simulink model "Model_vmaRHTS_R2019b_statespace"  (R2023a)
settings: Solver=ode4  StartTime=0.0  StopTime=100  FixedStep=dt  RelTol=1e-3
undefined symbols (not defined in the file): a0, a1, a2, a3, a4, a5, a6, a7, A_cplant, A_G1, A_Gpd, AgN, alpha1, alpha2, B_cplant, B_G1, B_Gpd, C_cplant, C_G1, C_Gpd, C_phys_5dof, CNrt, Cren, D_cplant, D_G1, D_Gpd, Ds, dt, dv1, dv2, EQ_intensity, EQ_sw, FN, G1, Gcld, Gd1, Gnd_ss, Hs1, Hs2, j1, j2, k3, k4, k6, K_phys_5dof, KNbar_inv, Koo, Kot, Kren, lN, M_phys_5dof, MNrt, Mren, RNbar
libraries: slpidlib x4, sldrtlib x1, dspsrcs4 x1
settings Model: Creator=icu327  LastModifiedBy=liangyu
settings SolverCC: AlgebraicLoopSolver=TrustRegion
settings DataIOCC: SaveFormat=Array  ReturnWorkspaceOutputs=off
settings DebuggingCC: UnconnectedInputMsg=warning  UnconnectedOutputMsg=warning  UnconnectedLineMsg=warning  ArithmeticOperatorsInVariantConditions=warning
settings HardwareCC: ProdBitPerLong=64  ProdHWDeviceType=Intel->x86-64 (Linux 64)
settings ModelReferenceCC: EnableRefExpFcnMdlSchedulingChecks=on
settings SFSimCC: CustomCodeUndefinedFunction=UseInterfaceOnly
settings RTWCC: Description=Simulink Desktop Real-Time  SystemTargetFile=sldrt.tlc  TemplateMakefile=sldrt.tmf  RTWCompilerOptimization=on
settings CodeAppCC: MaxIdLength=95  StateflowObjectComments=on
settings SimulinkDesktopRealTimeCC: TargetLibSuffix=_sldrt.a  TargetPreCompLibLocation=C:\Program Files\MATLAB\R2023a\toolbox\sldrt\lib\win64

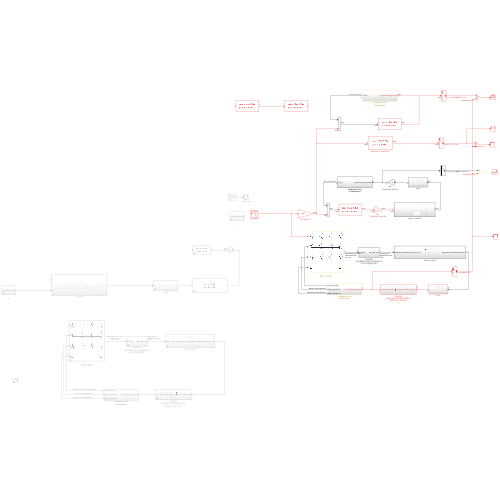
[thumbnail: Simulink's stored preview of the top-level diagram]
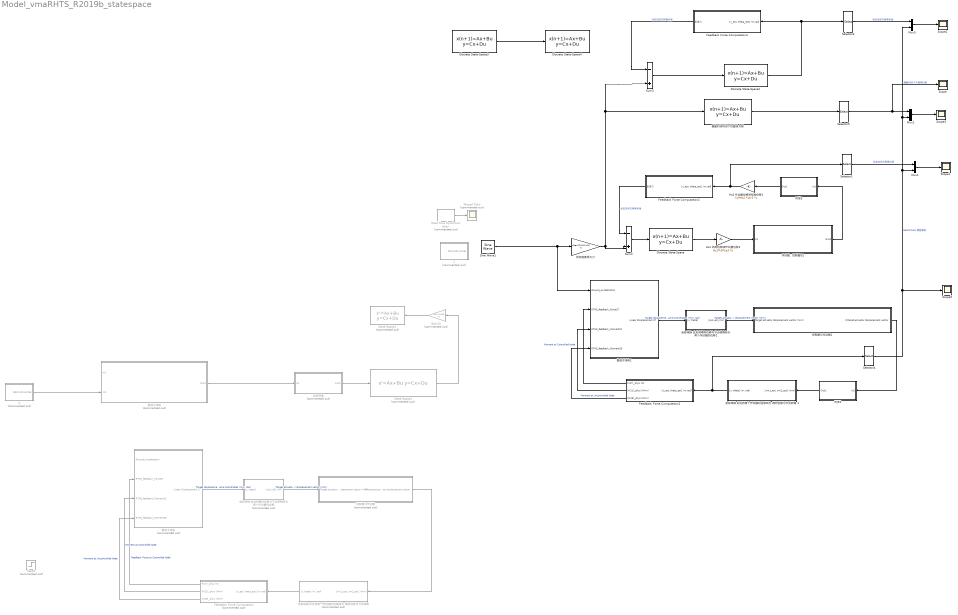
== system Model_vmaRHTS_R2019b_statespace ==
  " 2" : Subsystem  Commented=on
  " 4" : Subsystem  Commented=on
  " 数值子结构" : Subsystem  Commented=on
      mask Display: image('$imagefile'); % Use "Edit Image" on toolstrip to change.
  " 数值子结构1" : Subsystem
      mask Display: image('$imagefile'); % Use "Edit Image" on toolstrip to change.
  Discrete State-Space : DiscreteStateSpace  A=Gnd_ss.A  B=Gnd_ss.B  C=Gnd_ss.C  D=Gnd_ss.D  SampleTime=-1
  Discrete State-Space2 : DiscreteStateSpace  A=Gd1.A  B=Gd1.B  C=Gd1.C  D=Gd1.D  SampleTime=-1
  Discrete State-Space3 : DiscreteStateSpace  A=Gnd_ss.A  B=Gnd_ss.B  C=Gnd_ss.C  D=Gnd_ss.D  SampleTime=-1
  Discrete State-Space4 : DiscreteStateSpace  A=Ds.A  B=Ds.B  C=Ds.C  D=Ds.D  SampleTime=-1
  Feedback Force Computation : Subsystem  Commented=on
  Feedback Force Computation1 : Subsystem
  Feedback Force Computation2 : Subsystem
  Feedback Force Computation4 : Subsystem
  Gain10 : Gain  Commented=on  Gain=Hs2./1000  Multiplication=Matrix(K*u)
  Hs1 结构位移转作动器位移2 : Gain  Gain=Hs1*k6*1e3  Multiplication=Matrix(K*u)
  Hs2 作动器位移转结构位移1 : Gain  Gain=k4*Hs2.*1e-3  Multiplication=Matrix(K*u)
  Missed Ticks : Scope  Commented=on
  Mux1 : Mux  Inputs=2
  Mux2 : Mux  Inputs=2
  Mux3 : Mux  Inputs=2
  Real-Time Synchronization : sldrtlib/Real-Time Synchronization  Commented=on  SampleTime=dt  MaxMissedTicks=10000  ShowMissedTicks=on  YieldWhenWaiting=off
  Scope{,1..3,5} (5 alike) : Scope
  Selector1 : Selector  InputPortWidth=5  IndexOptions=Index vector (dialog)  Indices=[1]  OutputSizes=1
  Selector3 : Selector  InputPortWidth=5  IndexOptions=Index vector (dialog)  Indices=[1]  OutputSizes=1
  Selector4 : Selector  InputPortWidth=2  IndexOptions=Index vector (dialog)  Indices=[1]  OutputSizes=1
  Selector5 : Selector  InputPortWidth=5  IndexOptions=Index vector (dialog)  Indices=[1]  OutputSizes=1
  Sine Wave1 : dspsrcs4/Sine Wave  Amplitude=1  Frequency=1  Phase=0  SampleMode=Discrete  OutComplex=Real  CompMethod=Trigonometric fcn  TableSize=Speed  SampleTime=dt  SamplesPerFrame=1  ResetState=Restart at time zero  OutputFrames=off  dataType=double  wordLen=16  udDataType=sfix(16)  fracBitsMode=Best precision  numFracBits=15  OutDataTypeStr=double  LastOutDataTypeStr=double
  State-Space2 : StateSpace  Commented=on  A=A_G1  B=B_G1  C=C_G1  D=D_G1  InitialCondition=0
  State-Space3 : StateSpace  Commented=on  A=A_Gpd  B=B_Gpd  C=C_Gpd  D=D_Gpd  InitialCondition=0
  Step5 : Step  Commented=on  SampleTime=0
  Sum2 : Sum  Inputs=-|+
  Sum3 : Sum  Inputs=-|+
  作动器、控制器G1 : Subsystem
  坐标转换 : Subsystem  Commented=on
  "坐标转换 此处将两个作动器的位移转为 横向位移与节点转角 " : Subsystem  Commented=on
  坐标转换 此处将两个作动器的位移转为 横向位移与节点转角 1 : Subsystem
  坐标转换 此处将横向位移与节点转角转为 两个作动器的位移 : Subsystem  Commented=on
  坐标转换 此处将横向位移与节点转角转为 两个作动器的位移1 : Subsystem
  将加速度转为力 : Gain  Gain=-Mren*[1;0;1;1;0]  Multiplication=Matrix(K*u)
  控制器与作动器 : Subsystem  Commented=on
  控制器与作动器1 : Subsystem
  数值子结构 : Subsystem  Commented=on
  时滞2 : Subsystem
  时滞3 : Subsystem
  离散时间时间下的整体方程 : DiscreteStateSpace  A=Gcld.A  B=Gcld.B  C=Gcld.C  D=Gcld.D  SampleTime=-1
  wires:
  Feedback Force Computation/1(F(27)_phys (N)) -> " 数值子结构"/2(RTHS_feedback_Force27)  "Feedback Force at Controlled Node"
  Feedback Force Computation/3(M(29)_phys (N*m)) -> " 数值子结构"/4(RTHS_feedback_Moment29)  "Moment at Uncontrolled Node"
  "坐标转换 此处将两个作动器的位移转为 横向位移与节点转角 "/1("[x, theta] (m, rad)") -> Feedback Force Computation/1("[x_est, theta_est] (m,rad)")
  " 数值子结构"/1(Linear Displacement 27) -> 坐标转换 此处将横向位移与节点转角转为 两个作动器的位移/1("[x, theta]")  "Target displacement vector Frame coordinates (mm, rad)"
  Feedback Force Computation/2(M(21)_phys (N*m)) -> " 数值子结构"/3(RTHS_feedback_Moment21)  "Moment at Controlled Node"
  坐标转换 此处将横向位移与节点转角转为 两个作动器的位移/1("[xa1,xa2] mm") -> 控制器与作动器/1(Target actuator displacement vector (mm))  "Target actuator displacement vector (mm)"
  控制器与作动器/1(Filtered actuator displacement vector) -> "坐标转换 此处将两个作动器的位移转为 横向位移与节点转角 "/1("[xm1_est, xm2_est] (mm)")
  " 数值子结构1"/1(Linear Displacement 27) -> 坐标转换 此处将横向位移与节点转角转为 两个作动器的位移1/1("[x, theta]")  "Target displacement vector Frame coordinates (mm, rad)"
  坐标转换 此处将横向位移与节点转角转为 两个作动器的位移1/1("[xa1,xa2] mm") -> 控制器与作动器1/1(Target actuator displacement vector (mm))  "Target actuator displacement vector (mm)"
  Gain10/1 -> State-Space3/1
  State-Space2/1 -> Gain10/1
  " 4"/1(GROUND ACCEL) -> 数值子结构/2(In2)
  数值子结构/1(Out1) -> 坐标转换/1(In1)
  坐标转换/1(Out1) -> State-Space2/1
  Real-Time Synchronization/1 -> Missed Ticks/1
  Sine Wave1/1 -> " 数值子结构1"/1(Ground_Acceleration), 将加速度转为力/1
  Feedback Force Computation1/1(F(27)_phys (N)) -> " 数值子结构1"/2(RTHS_feedback_Force27)
  Feedback Force Computation1/2(M(21)_phys (N*m)) -> " 数值子结构1"/3(RTHS_feedback_Moment21)  "Moment at Controlled Node"
  Feedback Force Computation1/3(M(29)_phys (N*m)) -> " 数值子结构1"/4(RTHS_feedback_Moment29)  "Moment at Uncontrolled Node"
  Mux2/1 -> Scope3/1
  离散时间时间下的整体方程/1 -> Selector5/1
  Selector5/1 -> Scope/1, Mux2/1  "离散时间下方程等价版"
  控制器与作动器1/1(Filtered actuator displacement vector) -> 时滞2/1(In1)
  坐标转换 此处将两个作动器的位移转为 横向位移与节点转角 1/1("[x, theta] (m, rad)") -> Feedback Force Computation1/1("[x_est, theta_est] (m,rad)"), Selector4/1
  时滞2/1(Out1) -> 坐标转换 此处将两个作动器的位移转为 横向位移与节点转角 1/1("[xm1_est, xm2_est] (mm)")
  将加速度转为力/1 -> Sum3/2, 离散时间时间下的整体方程/1, Sum2/2
  作动器、控制器G1/1(Out1) -> 时滞3/1(In1)
  Feedback Force Computation2/1(反馈力) -> Sum2/1  "状态空间方程等价版"
  Hs2 作动器位移转结构位移1/1 -> Selector1/1, Feedback Force Computation2/1("[x_est, theta_est] (m,rad)")
  Discrete State-Space/1 -> Hs1 结构位移转作动器位移2/1
  时滞3/1(Out1) -> Hs2 作动器位移转结构位移1/1
  Sum2/1 -> Discrete State-Space/1
  Hs1 结构位移转作动器位移2/1 -> 作动器、控制器G1/1(In1)
  Selector1/1 -> Mux1/1  "状态空间方程等价版"
  Mux1/1 -> Scope1/1
  Mux3/1 -> Scope2/1
  Sum3/1 -> Discrete State-Space2/1
  Selector4/1 -> Mux3/2, Mux2/2, Mux1/2, Scope5/1  "benchmark模型原版"
  Selector3/1 -> Mux3/1  "状态空间方程等价版"
  Feedback Force Computation4/1(反馈力) -> Sum3/1  "状态空间方程等价版"
  Discrete State-Space2/1 -> Feedback Force Computation4/1("[x_est, theta_est] (m,rad)"), Selector3/1
  Discrete State-Space3/1 -> Discrete State-Space4/1

== system Model_vmaRHTS_R2019b_statespace/ 2 ==
  note: Benchmark Control Problem for
      | Multi-axial Real-time Hybrid Simulation
      | Ground Acceleration
  Clock : Clock
  EQ scaling factor : Gain  Gain=EQ_intensity  Multiplication=Matrix(K*u)
  GROUND ACCELERATION : ToWorkspace  VariableName=EQ_input  SampleTime=-1
      settings: Save2DSignal=2-D array (concatenate along first dimension)
  Ground motion record : Subsystem
  Multiport Switch : MultiPortSwitch  SaturateOnIntegerOverflow=off  InputSameDT=off
  SWITCH CONSTANT : Constant  Value=EQ_sw
  To Workspace : ToWorkspace  VariableName=t  SampleTime=dt
  GROUND ACCEL : Outport  VectorParamsAs1DForOutWhenUnconnected=off
  wires:
  Multiport Switch/1 -> EQ scaling factor/1
  EQ scaling factor/1 -> GROUND ACCELERATION/1, GROUND ACCEL/1
  Ground motion record/1(El Centro) -> Multiport Switch/2
  Ground motion record/2(Kobe) -> Multiport Switch/3
  Ground motion record/3(Morgan) -> Multiport Switch/4
  SWITCH CONSTANT/1 -> Multiport Switch/1
  Clock/1 -> To Workspace/1

== system Model_vmaRHTS_R2019b_statespace/ 4 ==
  note: Benchmark Control Problem for
      | Multi-axial Real-time Hybrid Simulation
      | Ground Acceleration
  Clock : Clock
  EQ scaling factor : Gain  Gain=EQ_intensity  Multiplication=Matrix(K*u)
  GROUND ACCELERATION : ToWorkspace  VariableName=EQ_input  SampleTime=-1
      settings: Save2DSignal=2-D array (concatenate along first dimension)
  Ground motion record : Subsystem
  Multiport Switch : MultiPortSwitch  SaturateOnIntegerOverflow=off  InputSameDT=off
  SWITCH CONSTANT : Constant  Value=EQ_sw
  To Workspace : ToWorkspace  VariableName=t  SampleTime=dt
  GROUND ACCEL : Outport  VectorParamsAs1DForOutWhenUnconnected=off
  wires:
  Multiport Switch/1 -> EQ scaling factor/1
  EQ scaling factor/1 -> GROUND ACCELERATION/1, GROUND ACCEL/1
  Ground motion record/1(El Centro) -> Multiport Switch/2
  Ground motion record/2(Kobe) -> Multiport Switch/3
  Ground motion record/3(Morgan) -> Multiport Switch/4
  SWITCH CONSTANT/1 -> Multiport Switch/1
  Clock/1 -> To Workspace/1

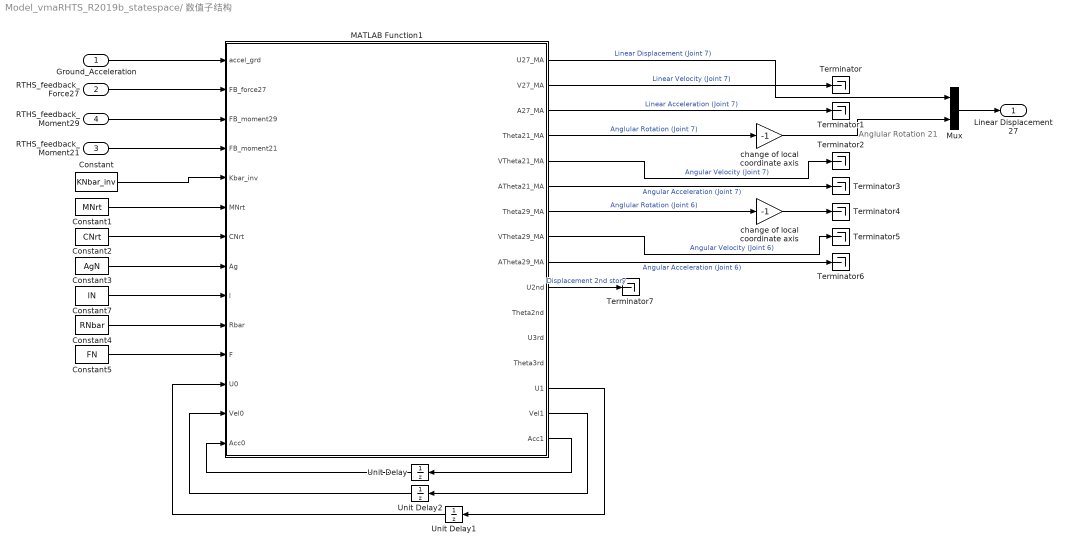
== system Model_vmaRHTS_R2019b_statespace/ 数值子结构 ==
  note: Anglular Rotation 21
  Ground_Acceleration : Inport
  RTHS_feedback_Force27 : Inport  Port=2
  RTHS_feedback_Moment21 : Inport  Port=3
  RTHS_feedback_Moment29 : Inport  Port=4
  Constant : Constant  Value=KNbar_inv  VectorParams1D=off
  Constant1 : Constant  Value=MNrt  VectorParams1D=off
  Constant2 : Constant  Value=CNrt  VectorParams1D=off
  Constant3 : Constant  Value=AgN  VectorParams1D=off
  Constant4 : Constant  Value=RNbar  VectorParams1D=off
  Constant5 : Constant  Value=FN  VectorParams1D=off
  Constant7 : Constant  Value=lN  VectorParams1D=off
  MATLAB Function1 : MATLAB Function  TreatAsAtomicUnit=on
  Mux : Mux  Inputs=2
  Terminator{,1..7} (8 alike) : Terminator
  Unit Delay : UnitDelay  SampleTime=-1  HasFrameUpgradeWarning=on
  Unit Delay1 : UnitDelay  SampleTime=-1  HasFrameUpgradeWarning=on
  Unit Delay2 : UnitDelay  SampleTime=-1  HasFrameUpgradeWarning=on
  change of local coordinate axis : Gain  Gain=-1
  "change of local coordinate axis  " : Gain  Gain=-1
  Linear Displacement 27 : Outport  VectorParamsAs1DForOutWhenUnconnected=off
  wires:
  Ground_Acceleration/1 -> MATLAB Function1/1(accel_grd)
  RTHS_feedback_Force27/1 -> MATLAB Function1/2(FB_force27)
  RTHS_feedback_Moment29/1 -> MATLAB Function1/3(FB_moment29)
  MATLAB Function1/1(U27_MA) -> Mux/1  "Linear Displacement (Joint 7)"
  MATLAB Function1/4(Theta21_MA) -> change of local coordinate axis/1  "Anglular Rotation (Joint 7)"
  Constant/1 -> MATLAB Function1/5(Kbar_inv)
  Constant1/1 -> MATLAB Function1/6(MNrt)
  Constant2/1 -> MATLAB Function1/7(CNrt)
  Constant3/1 -> MATLAB Function1/8(Ag)
  Constant7/1 -> MATLAB Function1/9(l)
  Constant4/1 -> MATLAB Function1/10(Rbar)
  Unit Delay1/1 -> MATLAB Function1/12(U0)
  Unit Delay2/1 -> MATLAB Function1/13(Vel0)
  Unit Delay/1 -> MATLAB Function1/14(Acc0)
  MATLAB Function1/15(Vel1) -> Unit Delay2/1
  MATLAB Function1/16(Acc1) -> Unit Delay/1
  MATLAB Function1/14(U1) -> Unit Delay1/1
  Constant5/1 -> MATLAB Function1/11(F)
  MATLAB Function1/2(V27_MA) -> Terminator/1  "Linear Velocity (Joint 7)"
  MATLAB Function1/3(A27_MA) -> Terminator1/1  "Linear Acceleration (Joint 7)"
  MATLAB Function1/5(VTheta21_MA) -> Terminator2/1  "Angular Velocity (Joint 7)"
  MATLAB Function1/6(ATheta21_MA) -> Terminator3/1  "Angular Acceleration (Joint 7)"
  MATLAB Function1/9(ATheta29_MA) -> Terminator6/1  "Angular Acceleration (Joint 6)"
  MATLAB Function1/8(VTheta29_MA) -> Terminator5/1  "Angular Velocity (Joint 6)"
  MATLAB Function1/7(Theta29_MA) -> "change of local coordinate axis  "/1  "Anglular Rotation (Joint 6)"
  RTHS_feedback_Moment21/1 -> MATLAB Function1/4(FB_moment21)
  change of local coordinate axis/1 -> Mux/2
  "change of local coordinate axis  "/1 -> Terminator4/1
  Mux/1 -> Linear Displacement 27/1
  MATLAB Function1/10(U2nd) -> Terminator7/1  "Displacement 2nd story"

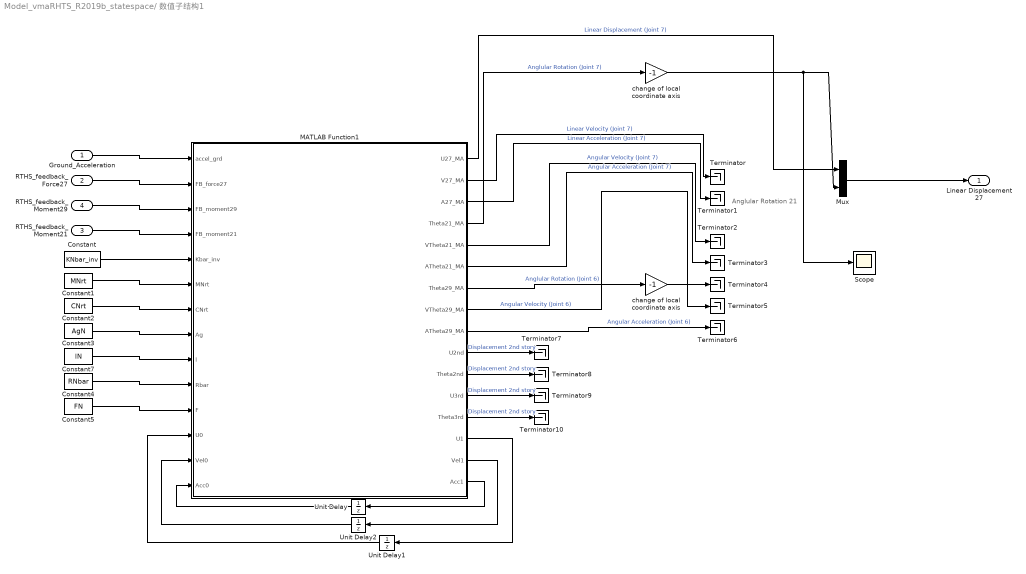
== system Model_vmaRHTS_R2019b_statespace/ 数值子结构1 ==
  note: Anglular Rotation 21
  Ground_Acceleration : Inport
  RTHS_feedback_Force27 : Inport  Port=2
  RTHS_feedback_Moment21 : Inport  Port=3
  RTHS_feedback_Moment29 : Inport  Port=4
  Constant : Constant  Value=KNbar_inv  VectorParams1D=off
  Constant1 : Constant  Value=MNrt  VectorParams1D=off
  Constant2 : Constant  Value=CNrt  VectorParams1D=off
  Constant3 : Constant  Value=AgN  VectorParams1D=off
  Constant4 : Constant  Value=RNbar  VectorParams1D=off
  Constant5 : Constant  Value=FN  VectorParams1D=off
  Constant7 : Constant  Value=lN  VectorParams1D=off
  MATLAB Function1 : MATLAB Function  TreatAsAtomicUnit=on
  Mux : Mux  Inputs=2
  Scope : Scope
  Terminator{,1..10} (11 alike) : Terminator
  Unit Delay : UnitDelay  SampleTime=-1  HasFrameUpgradeWarning=on
  Unit Delay1 : UnitDelay  SampleTime=-1  HasFrameUpgradeWarning=on
  Unit Delay2 : UnitDelay  SampleTime=-1  HasFrameUpgradeWarning=on
  change of local coordinate axis : Gain  Gain=-1
  "change of local coordinate axis  " : Gain  Gain=-1
  Linear Displacement 27 : Outport  VectorParamsAs1DForOutWhenUnconnected=off
  wires:
  Ground_Acceleration/1 -> MATLAB Function1/1(accel_grd)
  RTHS_feedback_Force27/1 -> MATLAB Function1/2(FB_force27)
  RTHS_feedback_Moment29/1 -> MATLAB Function1/3(FB_moment29)
  MATLAB Function1/1(U27_MA) -> Mux/1  "Linear Displacement (Joint 7)"
  MATLAB Function1/4(Theta21_MA) -> change of local coordinate axis/1  "Anglular Rotation (Joint 7)"
  Constant/1 -> MATLAB Function1/5(Kbar_inv)
  Constant1/1 -> MATLAB Function1/6(MNrt)
  Constant2/1 -> MATLAB Function1/7(CNrt)
  Constant3/1 -> MATLAB Function1/8(Ag)
  Constant7/1 -> MATLAB Function1/9(l)
  Constant4/1 -> MATLAB Function1/10(Rbar)
  Unit Delay1/1 -> MATLAB Function1/12(U0)
  Unit Delay2/1 -> MATLAB Function1/13(Vel0)
  Unit Delay/1 -> MATLAB Function1/14(Acc0)
  MATLAB Function1/15(Vel1) -> Unit Delay2/1
  MATLAB Function1/16(Acc1) -> Unit Delay/1
  MATLAB Function1/14(U1) -> Unit Delay1/1
  Constant5/1 -> MATLAB Function1/11(F)
  MATLAB Function1/2(V27_MA) -> Terminator/1  "Linear Velocity (Joint 7)"
  MATLAB Function1/3(A27_MA) -> Terminator1/1  "Linear Acceleration (Joint 7)"
  MATLAB Function1/5(VTheta21_MA) -> Terminator2/1  "Angular Velocity (Joint 7)"
  MATLAB Function1/6(ATheta21_MA) -> Terminator3/1  "Angular Acceleration (Joint 7)"
  MATLAB Function1/9(ATheta29_MA) -> Terminator6/1  "Angular Acceleration (Joint 6)"
  MATLAB Function1/8(VTheta29_MA) -> Terminator5/1  "Angular Velocity (Joint 6)"
  MATLAB Function1/7(Theta29_MA) -> "change of local coordinate axis  "/1  "Anglular Rotation (Joint 6)"
  RTHS_feedback_Moment21/1 -> MATLAB Function1/4(FB_moment21)
  change of local coordinate axis/1 -> Scope/1, Mux/2
  "change of local coordinate axis  "/1 -> Terminator4/1
  Mux/1 -> Linear Displacement 27/1
  MATLAB Function1/10(U2nd) -> Terminator7/1  "Displacement 2nd story"
  MATLAB Function1/11(Theta2nd) -> Terminator8/1  "Displacement 2nd story"
  MATLAB Function1/12(U3rd) -> Terminator9/1  "Displacement 2nd story"
  MATLAB Function1/13(Theta3rd) -> Terminator10/1  "Displacement 2nd story"

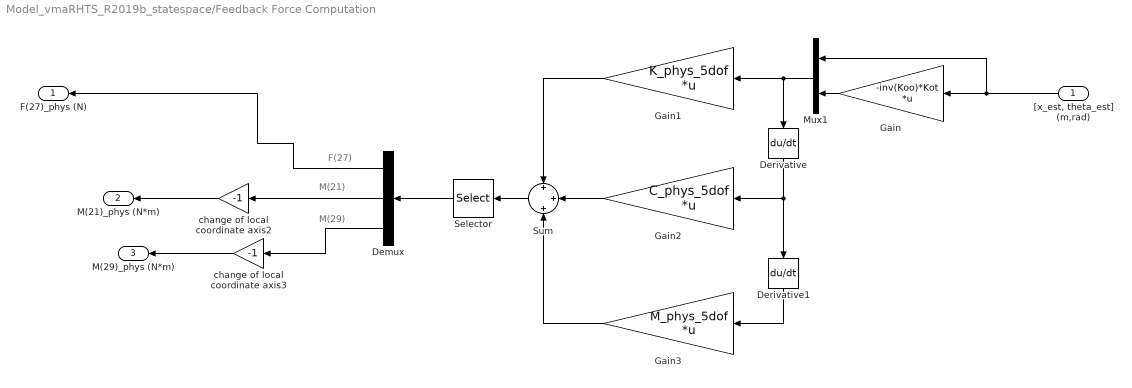
== system Model_vmaRHTS_R2019b_statespace/Feedback Force Computation ==
  note: F(27)
  note: M(21)
  note: M(29)
  "[x_est, theta_est] (m,rad)" : Inport
  Demux : Demux  Outputs=3
  Derivative : Derivative
  Derivative1 : Derivative
  Gain : Gain  Gain=-inv(Koo)*Kot  Multiplication=Matrix(K*u) (u vector)
  Gain1 : Gain  Gain=K_phys_5dof  Multiplication=Matrix(K*u) (u vector)
  Gain2 : Gain  Gain=C_phys_5dof  Multiplication=Matrix(K*u) (u vector)
  Gain3 : Gain  Gain=M_phys_5dof  Multiplication=Matrix(K*u) (u vector)
  Mux1 : Mux  Inputs=2
  Selector : Selector  InputPortWidth=5  IndexOptions=Index vector (dialog)  Indices=[1 2 3]  OutputSizes=1
  Sum : Sum  Inputs=+|+|+
  change of local coordinate axis2 : Gain  Gain=-1
  change of local coordinate axis3 : Gain  Gain=-1
  F(27)_phys (N) : Outport  VectorParamsAs1DForOutWhenUnconnected=off
  M(21)_phys (N*m) : Outport  Port=2  VectorParamsAs1DForOutWhenUnconnected=off
  M(29)_phys (N*m) : Outport  Port=3  VectorParamsAs1DForOutWhenUnconnected=off
  wires:
  Gain/1 -> Mux1/2
  Derivative1/1 -> Gain3/1
  Gain2/1 -> Sum/2
  Derivative/1 -> Gain2/1, Derivative1/1
  Gain1/1 -> Sum/1
  "[x_est, theta_est] (m,rad)"/1 -> Gain/1, Mux1/1
  Demux/1 -> F(27)_phys (N)/1
  Sum/1 -> Selector/1
  Selector/1 -> Demux/1
  Gain3/1 -> Sum/3
  Demux/2 -> change of local coordinate axis2/1
  Demux/3 -> change of local coordinate axis3/1
  Mux1/1 -> Derivative/1, Gain1/1
  change of local coordinate axis2/1 -> M(21)_phys (N*m)/1
  change of local coordinate axis3/1 -> M(29)_phys (N*m)/1

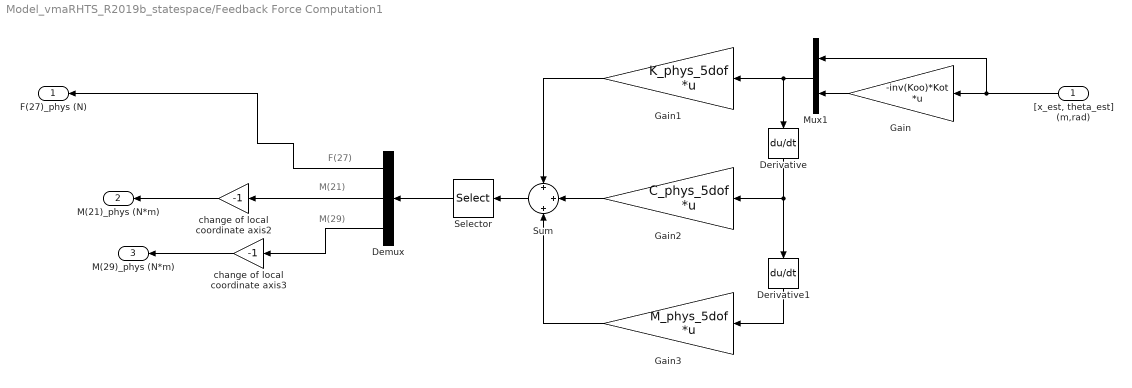
== system Model_vmaRHTS_R2019b_statespace/Feedback Force Computation1 ==
  note: F(27)
  note: M(21)
  note: M(29)
  "[x_est, theta_est] (m,rad)" : Inport
  Demux : Demux  Outputs=3
  Derivative : Derivative
  Derivative1 : Derivative
  Gain : Gain  Gain=-inv(Koo)*Kot  Multiplication=Matrix(K*u) (u vector)
  Gain1 : Gain  Gain=K_phys_5dof  Multiplication=Matrix(K*u) (u vector)
  Gain2 : Gain  Gain=C_phys_5dof  Multiplication=Matrix(K*u) (u vector)
  Gain3 : Gain  Gain=M_phys_5dof  Multiplication=Matrix(K*u) (u vector)
  Mux1 : Mux  Inputs=2
  Selector : Selector  InputPortWidth=5  IndexOptions=Index vector (dialog)  Indices=[1 2 3]  OutputSizes=1
  Sum : Sum  Inputs=+|+|+
  change of local coordinate axis2 : Gain  Gain=-1
  change of local coordinate axis3 : Gain  Gain=-1
  F(27)_phys (N) : Outport  VectorParamsAs1DForOutWhenUnconnected=off
  M(21)_phys (N*m) : Outport  Port=2  VectorParamsAs1DForOutWhenUnconnected=off
  M(29)_phys (N*m) : Outport  Port=3  VectorParamsAs1DForOutWhenUnconnected=off
  wires:
  Gain/1 -> Mux1/2
  Derivative1/1 -> Gain3/1
  Gain2/1 -> Sum/2
  Derivative/1 -> Gain2/1, Derivative1/1
  Gain1/1 -> Sum/1
  "[x_est, theta_est] (m,rad)"/1 -> Gain/1, Mux1/1
  Demux/1 -> F(27)_phys (N)/1
  Sum/1 -> Selector/1
  Selector/1 -> Demux/1
  Gain3/1 -> Sum/3
  Demux/2 -> change of local coordinate axis2/1
  Demux/3 -> change of local coordinate axis3/1
  Mux1/1 -> Derivative/1, Gain1/1
  change of local coordinate axis2/1 -> M(21)_phys (N*m)/1
  change of local coordinate axis3/1 -> M(29)_phys (N*m)/1

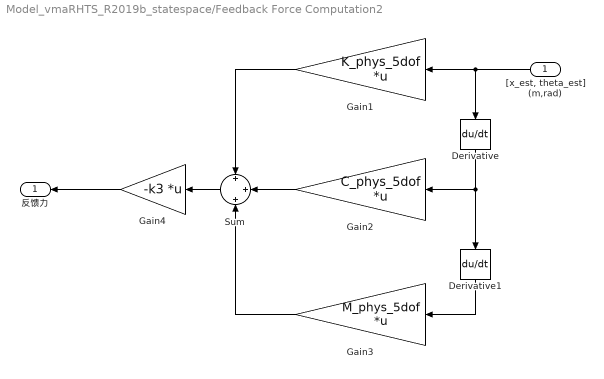
== system Model_vmaRHTS_R2019b_statespace/Feedback Force Computation2 ==
  "[x_est, theta_est] (m,rad)" : Inport
  Derivative : Derivative
  Derivative1 : Derivative
  Gain1 : Gain  Gain=K_phys_5dof  Multiplication=Matrix(K*u) (u vector)
  Gain2 : Gain  Gain=C_phys_5dof  Multiplication=Matrix(K*u) (u vector)
  Gain3 : Gain  Gain=M_phys_5dof  Multiplication=Matrix(K*u) (u vector)
  Gain4 : Gain  Gain=-k3  Multiplication=Matrix(K*u)
  Sum : Sum  Inputs=+|+|+
  反馈力 : Outport  VectorParamsAs1DForOutWhenUnconnected=off
  wires:
  Derivative1/1 -> Gain3/1
  Gain2/1 -> Sum/2
  Derivative/1 -> Gain2/1, Derivative1/1
  Gain1/1 -> Sum/1
  "[x_est, theta_est] (m,rad)"/1 -> Derivative/1, Gain1/1
  Sum/1 -> Gain4/1
  Gain3/1 -> Sum/3
  Gain4/1 -> 反馈力/1

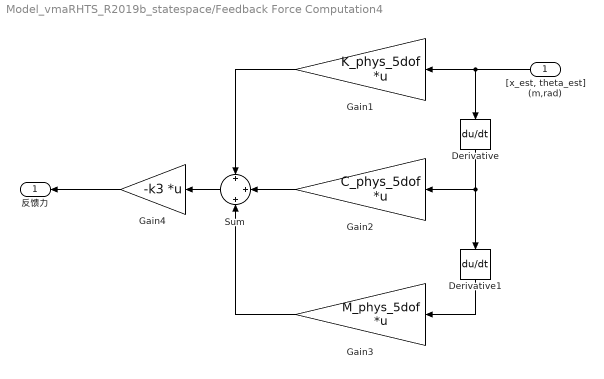
== system Model_vmaRHTS_R2019b_statespace/Feedback Force Computation4 ==
  "[x_est, theta_est] (m,rad)" : Inport
  Derivative : Derivative
  Derivative1 : Derivative
  Gain1 : Gain  Gain=K_phys_5dof  Multiplication=Matrix(K*u) (u vector)
  Gain2 : Gain  Gain=C_phys_5dof  Multiplication=Matrix(K*u) (u vector)
  Gain3 : Gain  Gain=M_phys_5dof  Multiplication=Matrix(K*u) (u vector)
  Gain4 : Gain  Gain=-k3  Multiplication=Matrix(K*u)
  Sum : Sum  Inputs=+|+|+
  反馈力 : Outport  VectorParamsAs1DForOutWhenUnconnected=off
  wires:
  Derivative1/1 -> Gain3/1
  Gain2/1 -> Sum/2
  Derivative/1 -> Gain2/1, Derivative1/1
  Gain1/1 -> Sum/1
  "[x_est, theta_est] (m,rad)"/1 -> Derivative/1, Gain1/1
  Sum/1 -> Gain4/1
  Gain3/1 -> Sum/3
  Gain4/1 -> 反馈力/1

== system Model_vmaRHTS_R2019b_statespace/作动器、控制器G1 ==
  In1 : Inport
  State-Space : StateSpace  A=G1.A  B=G1.B  C=G1.C  D=G1.D  InitialCondition=0
  Out1 : Outport
  wires:
  State-Space/1 -> Out1/1
  In1/1 -> State-Space/1

== system Model_vmaRHTS_R2019b_statespace/坐标转换 ==
  In1 : Inport
  Gain8 : Gain  Commented=on  Gain=k6  Multiplication=Matrix(K*u)
  Gain9 : Gain  Commented=on  Gain=Hs1.*1000  Multiplication=Matrix(K*u)
  Out1 : Outport
  wires:
  Gain8/1 -> Gain9/1
  In1/1 -> Gain8/1
  Gain9/1 -> Out1/1

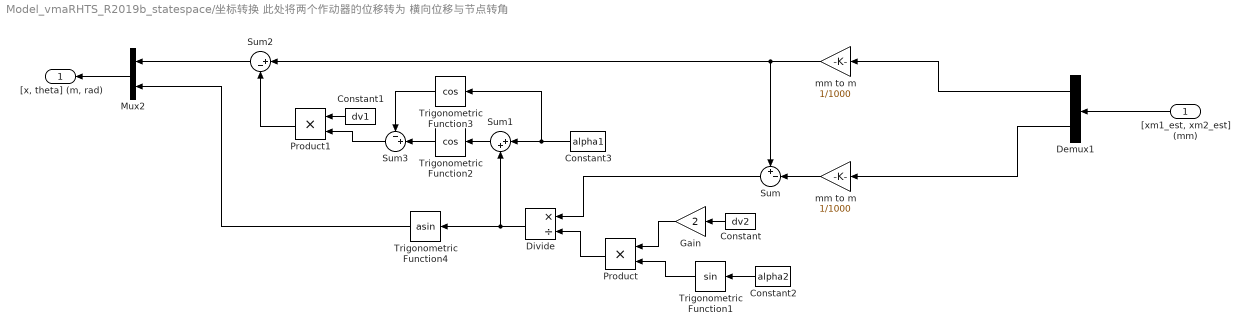
== system Model_vmaRHTS_R2019b_statespace/坐标转换 此处将两个作动器的位移转为 横向位移与节点转角  ==
  "[xm1_est, xm2_est] (mm)" : Inport
  Constant : Constant  Value=dv2
  Constant1 : Constant  Value=dv1
  Constant2 : Constant  Value=alpha2
  Constant3 : Constant  Value=alpha1
  Demux1 : Demux  Outputs=2
  Divide : Product  Inputs=*/
  Gain : Gain  Gain=2
  Mux2 : Mux  Inputs=2
  Product : Product
  Product1 : Product
  Sum : Sum  Inputs=+-|
  Sum1 : Sum  Inputs=|++
  Sum2 : Sum  Inputs=|+-
  Sum3 : Sum  Inputs=-+|
  Trigonometric Function1 : Trigonometry
  Trigonometric Function2 : Trigonometry  Operator=cos
  Trigonometric Function3 : Trigonometry  Operator=cos
  Trigonometric Function4 : Trigonometry  Operator=asin
  mm to m : Gain  Gain=1/1000
  "mm to m " : Gain  Gain=1/1000
  "[x, theta] (m, rad)" : Outport  VectorParamsAs1DForOutWhenUnconnected=off
  wires:
  Constant2/1 -> Trigonometric Function1/1
  Constant1/1 -> Product1/1
  Demux1/1 -> mm to m/1
  Demux1/2 -> "mm to m "/1
  Sum/1 -> Divide/1
  Constant/1 -> Gain/1
  Trigonometric Function1/1 -> Product/2
  Gain/1 -> Product/1
  Product/1 -> Divide/2
  Divide/1 -> Sum1/2, Trigonometric Function4/1
  Sum1/1 -> Trigonometric Function2/1
  Constant3/1 -> Sum1/1, Trigonometric Function3/1
  Sum3/1 -> Product1/2
  Sum2/1 -> Mux2/1
  Trigonometric Function2/1 -> Sum3/2
  Trigonometric Function3/1 -> Sum3/1
  Product1/1 -> Sum2/2
  mm to m/1 -> Sum2/1, Sum/1
  "mm to m "/1 -> Sum/2
  Trigonometric Function4/1 -> Mux2/2
  "[xm1_est, xm2_est] (mm)"/1 -> Demux1/1
  Mux2/1 -> "[x, theta] (m, rad)"/1

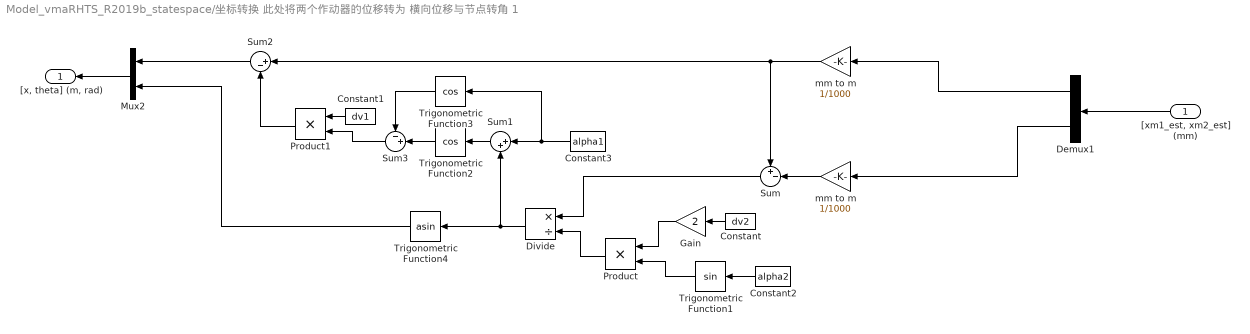
== system Model_vmaRHTS_R2019b_statespace/坐标转换 此处将两个作动器的位移转为 横向位移与节点转角 1 ==
  "[xm1_est, xm2_est] (mm)" : Inport
  Constant : Constant  Value=dv2
  Constant1 : Constant  Value=dv1
  Constant2 : Constant  Value=alpha2
  Constant3 : Constant  Value=alpha1
  Demux1 : Demux  Outputs=2
  Divide : Product  Inputs=*/
  Gain : Gain  Gain=2
  Mux2 : Mux  Inputs=2
  Product : Product
  Product1 : Product
  Sum : Sum  Inputs=+-|
  Sum1 : Sum  Inputs=|++
  Sum2 : Sum  Inputs=|+-
  Sum3 : Sum  Inputs=-+|
  Trigonometric Function1 : Trigonometry
  Trigonometric Function2 : Trigonometry  Operator=cos
  Trigonometric Function3 : Trigonometry  Operator=cos
  Trigonometric Function4 : Trigonometry  Operator=asin
  mm to m : Gain  Gain=1/1000
  "mm to m " : Gain  Gain=1/1000
  "[x, theta] (m, rad)" : Outport  VectorParamsAs1DForOutWhenUnconnected=off
  wires:
  Constant2/1 -> Trigonometric Function1/1
  Constant1/1 -> Product1/1
  Demux1/1 -> mm to m/1
  Demux1/2 -> "mm to m "/1
  Sum/1 -> Divide/1
  Constant/1 -> Gain/1
  Trigonometric Function1/1 -> Product/2
  Gain/1 -> Product/1
  Product/1 -> Divide/2
  Divide/1 -> Sum1/2, Trigonometric Function4/1
  Sum1/1 -> Trigonometric Function2/1
  Constant3/1 -> Sum1/1, Trigonometric Function3/1
  Sum3/1 -> Product1/2
  Sum2/1 -> Mux2/1
  Trigonometric Function2/1 -> Sum3/2
  Trigonometric Function3/1 -> Sum3/1
  Product1/1 -> Sum2/2
  mm to m/1 -> Sum2/1, Sum/1
  "mm to m "/1 -> Sum/2
  Trigonometric Function4/1 -> Mux2/2
  "[xm1_est, xm2_est] (mm)"/1 -> Demux1/1
  Mux2/1 -> "[x, theta] (m, rad)"/1

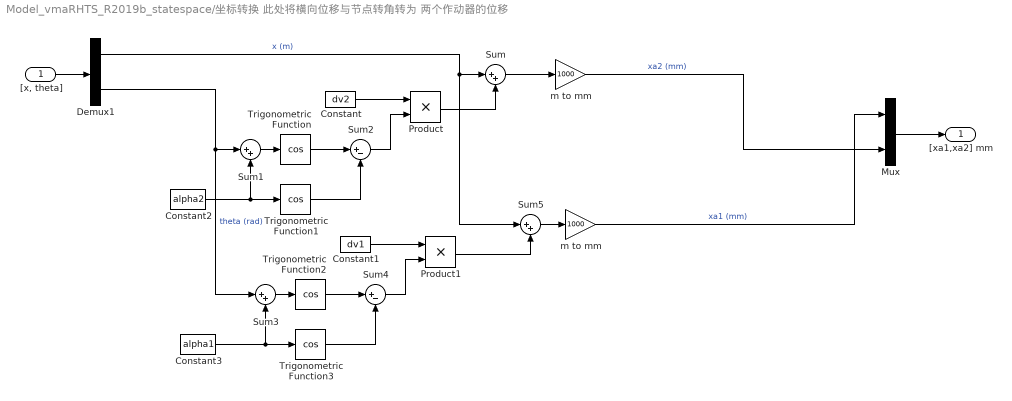
== system Model_vmaRHTS_R2019b_statespace/坐标转换 此处将横向位移与节点转角转为 两个作动器的位移 ==
  "[x, theta]" : Inport
  Constant : Constant  Value=dv2
  Constant1 : Constant  Value=dv1
  Constant2 : Constant  Value=alpha2
  Constant3 : Constant  Value=alpha1
  Demux1 : Demux  Outputs=2
  Mux : Mux  Inputs=2
  Product : Product
  Product1 : Product
  Sum{,1,3,5} (4 alike) : Sum  Inputs=|++
  Sum2 : Sum  Inputs=|+-
  Sum4 : Sum  Inputs=|+-
  Trigonometric Function{,1..3} (4 alike) : Trigonometry  Operator=cos
  m to mm : Gain  Gain=1000
  "m to mm " : Gain  Gain=1000
  "[xa1,xa2] mm" : Outport  VectorParamsAs1DForOutWhenUnconnected=off
  wires:
  Constant/1 -> Product/1
  Constant2/1 -> Sum1/2, Trigonometric Function1/1
  Sum1/1 -> Trigonometric Function/1
  Trigonometric Function/1 -> Sum2/1
  Trigonometric Function1/1 -> Sum2/2
  Sum2/1 -> Product/2
  Product/1 -> Sum/2
  Sum/1 -> m to mm/1
  Sum4/1 -> Product1/2
  Trigonometric Function3/1 -> Sum4/2
  Trigonometric Function2/1 -> Sum4/1
  Sum3/1 -> Trigonometric Function2/1
  Constant3/1 -> Sum3/2, Trigonometric Function3/1
  Constant1/1 -> Product1/1
  Product1/1 -> Sum5/2
  Sum5/1 -> "m to mm "/1
  "m to mm "/1 -> Mux/1  "xa1 (mm)"
  m to mm/1 -> Mux/2  "xa2 (mm)"
  Demux1/1 -> Sum/1, Sum5/1  "x (m)"
  "[x, theta]"/1 -> Demux1/1
  Demux1/2 -> Sum3/1, Sum1/1  "theta (rad)"
  Mux/1 -> "[xa1,xa2] mm"/1

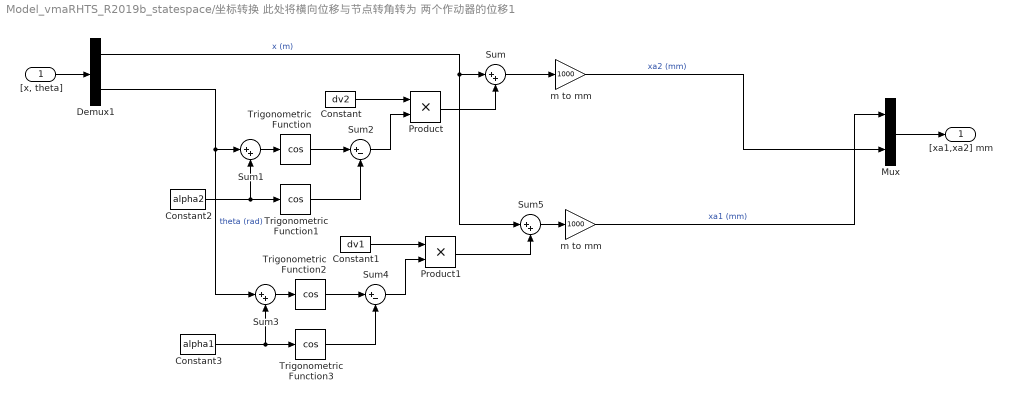
== system Model_vmaRHTS_R2019b_statespace/坐标转换 此处将横向位移与节点转角转为 两个作动器的位移1 ==
  "[x, theta]" : Inport
  Constant : Constant  Value=dv2
  Constant1 : Constant  Value=dv1
  Constant2 : Constant  Value=alpha2
  Constant3 : Constant  Value=alpha1
  Demux1 : Demux  Outputs=2
  Mux : Mux  Inputs=2
  Product : Product
  Product1 : Product
  Sum{,1,3,5} (4 alike) : Sum  Inputs=|++
  Sum2 : Sum  Inputs=|+-
  Sum4 : Sum  Inputs=|+-
  Trigonometric Function{,1..3} (4 alike) : Trigonometry  Operator=cos
  m to mm : Gain  Gain=1000
  "m to mm " : Gain  Gain=1000
  "[xa1,xa2] mm" : Outport  VectorParamsAs1DForOutWhenUnconnected=off
  wires:
  Constant/1 -> Product/1
  Constant2/1 -> Sum1/2, Trigonometric Function1/1
  Sum1/1 -> Trigonometric Function/1
  Trigonometric Function/1 -> Sum2/1
  Trigonometric Function1/1 -> Sum2/2
  Sum2/1 -> Product/2
  Product/1 -> Sum/2
  Sum/1 -> m to mm/1
  Sum4/1 -> Product1/2
  Trigonometric Function3/1 -> Sum4/2
  Trigonometric Function2/1 -> Sum4/1
  Sum3/1 -> Trigonometric Function2/1
  Constant3/1 -> Sum3/2, Trigonometric Function3/1
  Constant1/1 -> Product1/1
  Product1/1 -> Sum5/2
  Sum5/1 -> "m to mm "/1
  "m to mm "/1 -> Mux/1  "xa1 (mm)"
  m to mm/1 -> Mux/2  "xa2 (mm)"
  Demux1/1 -> Sum/1, Sum5/1  "x (m)"
  "[x, theta]"/1 -> Demux1/1
  Demux1/2 -> Sum3/1, Sum1/1  "theta (rad)"
  Mux/1 -> "[xa1,xa2] mm"/1

== system Model_vmaRHTS_R2019b_statespace/控制器与作动器 ==
  Target actuator displacement vector (mm) : Inport
  Control Plant4 : StateSpace  A=A_cplant  B=B_cplant  C=C_cplant  D=D_cplant  InitialCondition=0
  Demux7 : Demux  Outputs=2
  Mux4 : Mux  Inputs=2
  PID Controller2 : slpidlib/PID Controller  Controller=PID  Form=Parallel  TimeDomain=Discrete-time  UseExternalTs=off  SampleTime=-1  IntegratorMethod=Forward Euler  FilterMethod=Forward Euler  ControllerParametersSource=internal  P=1  I=50  UseKiTs=off  D=1e-10  N=100  UseFilter=off  TunerSelectOption=Transfer Function Based (PID Tuner App)  InitialConditionSource=internal  InitialConditionForIntegrator=0  InitialConditionForFilter=0  DifferentiatorICPrevScaledInput=0  ExternalReset=none  TrackingMode=off  Kt=1  LimitOutput=off  SatLimitsSource=internal  UpperSaturationLimit=inf  LowerSaturationLimit=-inf  LinearizeAsGain=on  AntiWindupMode=none  Kb=1  LimitIntegrator=off  UpperIntegratorSaturationLimit=inf  LowerIntegratorSaturationLimit=-inf  POutMin=[]  POutMax=[]  IOutMin=[]  IOutMax=[]  DOutMin=[]  DOutMax=[]  NOutMin=[]  NOutMax=[]  SumOutMin=[]  SumOutMax=[]  SaturationOutMin=[]  SaturationOutMax=[]  PParamMin=[]  PParamMax=[]  IParamMin=[]  IParamMax=[]  DParamMin=[]  DParamMax=[]  NParamMin=[]  NParamMax=[]  KbParamMin=[]  KbParamMax=[]  KtParamMin=[]  KtParamMax=[]  KbOutMin=[]  KbOutMax=[]  KtOutMin=[]  KtOutMax=[]  IntegratorOutMin=[]  IntegratorOutMax=[]  FilterOutMin=[]  FilterOutMax=[]  SumI1OutMin=[]  SumI1OutMax=[]  SumI2OutMin=[]  SumI2OutMax=[]  SumI3OutMin=[]  SumI3OutMax=[]  SumI4OutMin=[]  SumI4OutMax=[]  SumDOutMin=[]  SumDOutMax=[]  DifferentiatorOutMin=[]  DifferentiatorOutMax=[]  FilterDiffOutCoefMin=[]  FilterDiffOutCoefMax=[]  ReciprocalOutMin=[]  ReciprocalOutMax=[]  SumDenOutMin=[]  SumDenOutMax=[]  SumNumOutMin=[]  SumNumOutMax=[]  DivideOutMin=[]  DivideOutMax=[]  UdiffTsProdOutMin=[]  UdiffTsProdOutMax=[]  NTsProdOutMin=[]  NTsProdOutMax=[]  UintegralTsProdOutMin=[]  UintegralTsProdOutMax=[]  UngainTsProdOutMin=[]  UngainTsProdOutMax=[]  ClampingZeroOutDataTypeStr=Inherit: Inherit via back propagation  ClampingZeroOutMin=[]  ClampingZeroOutMax=[]  FilterDenConstantOutDataTypeStr=Inherit: Inherit via back propagation  FilterDenConstantOutMin=[]  FilterDenConstantOutMax=[]  PCopyOutDataTypeStr=Inherit: Inherit via back propagation  PCopyOutMin=[]  PCopyOutMax=[]  NCopyOutDataTypeStr=Inherit: Inherit via back propagation  NCopyOutMin=[]  NCopyOutMax=[]  IntegratorContinuousStateAttributes=''  IntegratorStateMustResolveToSignalObject=off  IntegratorRTWStateStorageClass=Auto  FilterContinuousStateAttributes=''  FilterStateMustResolveToSignalObject=off  FilterRTWStateStorageClass=Auto  ParallelPVariant=InternalParameters  IdealPVariant=Disabled  IVariant=InternalParameters  DVariant=InternalParameters  IntegratorVariant=Discrete  SatVariant=Disabled  AWVariant=Passthrough  PCopyVariant=Disabled  TRVariant=Disabled  FdbkBlocksVariant=Forward  IdealPFdbkVariant=Disabled  SatFdbkVariant=Disabled  DerivativeFilterVariant=Differentiator  NVariant=Passthrough  NCopyVariant=Disabled_SignalSpec  FilterICVariant=InternalICsDifferentiator  IntegratorICVariant=InternalICs  ExternalResetVariant=Disabled  TRSumVariant=Passthrough  SumFdbkVariant=Disabled  SumVariant=Sum_PID  TsampFilterVariant=InternalTs  TsampNgainVariant=Passthrough  TsampIntegralVariant=Disabled_SignalSpec  ExternalSaturationOutDataTypeStr=Inherit: Same as second input
  PID Controller4 : slpidlib/PID Controller  Controller=PID  Form=Parallel  TimeDomain=Discrete-time  UseExternalTs=off  SampleTime=-1  IntegratorMethod=Forward Euler  FilterMethod=Forward Euler  ControllerParametersSource=internal  P=1  I=50  UseKiTs=off  D=1e-10  N=100  UseFilter=on  TunerSelectOption=Transfer Function Based (PID Tuner App)  InitialConditionSource=internal  InitialConditionForIntegrator=0  InitialConditionForFilter=0  DifferentiatorICPrevScaledInput=0  ExternalReset=none  TrackingMode=off  Kt=1  LimitOutput=off  SatLimitsSource=internal  UpperSaturationLimit=inf  LowerSaturationLimit=-inf  LinearizeAsGain=on  AntiWindupMode=none  Kb=1  LimitIntegrator=off  UpperIntegratorSaturationLimit=inf  LowerIntegratorSaturationLimit=-inf  POutMin=[]  POutMax=[]  IOutMin=[]  IOutMax=[]  DOutMin=[]  DOutMax=[]  NOutMin=[]  NOutMax=[]  SumOutMin=[]  SumOutMax=[]  SaturationOutMin=[]  SaturationOutMax=[]  PParamMin=[]  PParamMax=[]  IParamMin=[]  IParamMax=[]  DParamMin=[]  DParamMax=[]  NParamMin=[]  NParamMax=[]  KbParamMin=[]  KbParamMax=[]  KtParamMin=[]  KtParamMax=[]  KbOutMin=[]  KbOutMax=[]  KtOutMin=[]  KtOutMax=[]  IntegratorOutMin=[]  IntegratorOutMax=[]  FilterOutMin=[]  FilterOutMax=[]  SumI1OutMin=[]  SumI1OutMax=[]  SumI2OutMin=[]  SumI2OutMax=[]  SumI3OutMin=[]  SumI3OutMax=[]  SumI4OutMin=[]  SumI4OutMax=[]  SumDOutMin=[]  SumDOutMax=[]  DifferentiatorOutMin=[]  DifferentiatorOutMax=[]  FilterDiffOutCoefMin=[]  FilterDiffOutCoefMax=[]  ReciprocalOutMin=[]  ReciprocalOutMax=[]  SumDenOutMin=[]  SumDenOutMax=[]  SumNumOutMin=[]  SumNumOutMax=[]  DivideOutMin=[]  DivideOutMax=[]  UdiffTsProdOutMin=[]  UdiffTsProdOutMax=[]  NTsProdOutMin=[]  NTsProdOutMax=[]  UintegralTsProdOutMin=[]  UintegralTsProdOutMax=[]  UngainTsProdOutMin=[]  UngainTsProdOutMax=[]  ClampingZeroOutDataTypeStr=Inherit: Inherit via back propagation  ClampingZeroOutMin=[]  ClampingZeroOutMax=[]  FilterDenConstantOutDataTypeStr=Inherit: Inherit via back propagation  FilterDenConstantOutMin=[]  FilterDenConstantOutMax=[]  PCopyOutDataTypeStr=Inherit: Inherit via back propagation  PCopyOutMin=[]  PCopyOutMax=[]  NCopyOutDataTypeStr=Inherit: Inherit via back propagation  NCopyOutMin=[]  NCopyOutMax=[]  IntegratorContinuousStateAttributes=''  IntegratorStateMustResolveToSignalObject=off  IntegratorRTWStateStorageClass=Auto  FilterContinuousStateAttributes=''  FilterStateMustResolveToSignalObject=off  FilterRTWStateStorageClass=Auto  ParallelPVariant=InternalParameters  IdealPVariant=Disabled  IVariant=InternalParameters  DVariant=InternalParameters  IntegratorVariant=Discrete  SatVariant=Disabled  AWVariant=Passthrough  PCopyVariant=Disabled  TRVariant=Disabled  FdbkBlocksVariant=Forward  IdealPFdbkVariant=Disabled  SatFdbkVariant=Disabled  DerivativeFilterVariant=ForwardEulerFilter  NVariant=InternalParameters  NCopyVariant=Disabled  FilterICVariant=InternalICsFilter  IntegratorICVariant=InternalICs  ExternalResetVariant=Disabled  TRSumVariant=Passthrough  SumFdbkVariant=Disabled  SumVariant=Sum_PID  TsampFilterVariant=InternalTs  TsampNgainVariant=Passthrough  TsampIntegralVariant=Disabled_SignalSpec  ExternalSaturationOutDataTypeStr=Inherit: Same as second input
  Sum11 : Sum  Inputs=|+-
  Filtered actuator displacement vector : Outport
  wires:
  PID Controller4/1 -> Mux4/2
  Control Plant4/1 -> Filtered actuator displacement vector/1, Sum11/2  "Filtered actuator displacement vector"
  Demux7/1 -> PID Controller2/1
  Sum11/1 -> Demux7/1
  PID Controller2/1 -> Mux4/1
  Mux4/1 -> Control Plant4/1
  Demux7/2 -> PID Controller4/1
  Target actuator displacement vector (mm)/1 -> Sum11/1

== system Model_vmaRHTS_R2019b_statespace/控制器与作动器1 ==
  Target actuator displacement vector (mm) : Inport
  Control Plant4 : StateSpace  A=A_cplant  B=B_cplant  C=C_cplant  D=D_cplant  InitialCondition=0
  Demux7 : Demux  Outputs=2
  Mux4 : Mux  Inputs=2
  PID Controller1 : slpidlib/PID Controller  Controller=PID  Form=Parallel  TimeDomain=Continuous-time  UseExternalTs=off  SampleTime=-1  IntegratorMethod=Forward Euler  FilterMethod=Forward Euler  ControllerParametersSource=internal  P=1.5  I=45  UseKiTs=off  D=1e-8  N=1000  UseFilter=on  TunerSelectOption=Transfer Function Based (PID Tuner App)  InitialConditionSource=internal  InitialConditionForIntegrator=0  InitialConditionForFilter=0  DifferentiatorICPrevScaledInput=0  ExternalReset=none  TrackingMode=off  Kt=1  LimitOutput=off  SatLimitsSource=internal  UpperSaturationLimit=inf  LowerSaturationLimit=-inf  LinearizeAsGain=on  AntiWindupMode=none  Kb=1  LimitIntegrator=off  UpperIntegratorSaturationLimit=inf  LowerIntegratorSaturationLimit=-inf  POutMin=[]  POutMax=[]  IOutMin=[]  IOutMax=[]  DOutMin=[]  DOutMax=[]  NOutMin=[]  NOutMax=[]  SumOutMin=[]  SumOutMax=[]  SaturationOutMin=[]  SaturationOutMax=[]  PParamMin=[]  PParamMax=[]  IParamMin=[]  IParamMax=[]  DParamMin=[]  DParamMax=[]  NParamMin=[]  NParamMax=[]  KbParamMin=[]  KbParamMax=[]  KtParamMin=[]  KtParamMax=[]  KbOutMin=[]  KbOutMax=[]  KtOutMin=[]  KtOutMax=[]  IntegratorOutMin=[]  IntegratorOutMax=[]  FilterOutMin=[]  FilterOutMax=[]  SumI1OutMin=[]  SumI1OutMax=[]  SumI2OutMin=[]  SumI2OutMax=[]  SumI3OutMin=[]  SumI3OutMax=[]  SumI4OutMin=[]  SumI4OutMax=[]  SumDOutMin=[]  SumDOutMax=[]  DifferentiatorOutMin=[]  DifferentiatorOutMax=[]  FilterDiffOutCoefMin=[]  FilterDiffOutCoefMax=[]  ReciprocalOutMin=[]  ReciprocalOutMax=[]  SumDenOutMin=[]  SumDenOutMax=[]  SumNumOutMin=[]  SumNumOutMax=[]  DivideOutMin=[]  DivideOutMax=[]  UdiffTsProdOutMin=[]  UdiffTsProdOutMax=[]  NTsProdOutMin=[]  NTsProdOutMax=[]  UintegralTsProdOutMin=[]  UintegralTsProdOutMax=[]  UngainTsProdOutMin=[]  UngainTsProdOutMax=[]  ClampingZeroOutDataTypeStr=Inherit: Inherit via back propagation  ClampingZeroOutMin=[]  ClampingZeroOutMax=[]  FilterDenConstantOutDataTypeStr=Inherit: Inherit via back propagation  FilterDenConstantOutMin=[]  FilterDenConstantOutMax=[]  PCopyOutDataTypeStr=Inherit: Inherit via back propagation  PCopyOutMin=[]  PCopyOutMax=[]  NCopyOutDataTypeStr=Inherit: Inherit via back propagation  NCopyOutMin=[]  NCopyOutMax=[]  IntegratorContinuousStateAttributes=''  IntegratorStateMustResolveToSignalObject=off  IntegratorRTWStateStorageClass=Auto  FilterContinuousStateAttributes=''  FilterStateMustResolveToSignalObject=off  FilterRTWStateStorageClass=Auto  ParallelPVariant=InternalParameters  IdealPVariant=Disabled  IVariant=InternalParameters  DVariant=InternalParameters  IntegratorVariant=Continuous  SatVariant=Disabled  AWVariant=Passthrough  PCopyVariant=Disabled  TRVariant=Disabled  FdbkBlocksVariant=Forward  IdealPFdbkVariant=Disabled  SatFdbkVariant=Disabled  DerivativeFilterVariant=ContFilter  NVariant=InternalParameters  NCopyVariant=Disabled  FilterICVariant=InternalICsFilter  IntegratorICVariant=InternalICs  ExternalResetVariant=Disabled  TRSumVariant=Passthrough  SumFdbkVariant=Disabled  SumVariant=Sum_PID  TsampFilterVariant=InternalTs  TsampNgainVariant=Passthrough  TsampIntegralVariant=Disabled_SignalSpec  ExternalSaturationOutDataTypeStr=Inherit: Same as second input
  PID Controller2 : slpidlib/PID Controller  Controller=PID  Form=Parallel  TimeDomain=Continuous-time  UseExternalTs=off  SampleTime=-1  IntegratorMethod=Forward Euler  FilterMethod=Forward Euler  ControllerParametersSource=internal  P=1.5  I=45  UseKiTs=off  D=1e-8  N=1000  UseFilter=on  TunerSelectOption=Transfer Function Based (PID Tuner App)  InitialConditionSource=internal  InitialConditionForIntegrator=0  InitialConditionForFilter=0  DifferentiatorICPrevScaledInput=0  ExternalReset=none  TrackingMode=off  Kt=1  LimitOutput=off  SatLimitsSource=internal  UpperSaturationLimit=inf  LowerSaturationLimit=-inf  LinearizeAsGain=on  AntiWindupMode=none  Kb=1  LimitIntegrator=off  UpperIntegratorSaturationLimit=inf  LowerIntegratorSaturationLimit=-inf  POutMin=[]  POutMax=[]  IOutMin=[]  IOutMax=[]  DOutMin=[]  DOutMax=[]  NOutMin=[]  NOutMax=[]  SumOutMin=[]  SumOutMax=[]  SaturationOutMin=[]  SaturationOutMax=[]  PParamMin=[]  PParamMax=[]  IParamMin=[]  IParamMax=[]  DParamMin=[]  DParamMax=[]  NParamMin=[]  NParamMax=[]  KbParamMin=[]  KbParamMax=[]  KtParamMin=[]  KtParamMax=[]  KbOutMin=[]  KbOutMax=[]  KtOutMin=[]  KtOutMax=[]  IntegratorOutMin=[]  IntegratorOutMax=[]  FilterOutMin=[]  FilterOutMax=[]  SumI1OutMin=[]  SumI1OutMax=[]  SumI2OutMin=[]  SumI2OutMax=[]  SumI3OutMin=[]  SumI3OutMax=[]  SumI4OutMin=[]  SumI4OutMax=[]  SumDOutMin=[]  SumDOutMax=[]  DifferentiatorOutMin=[]  DifferentiatorOutMax=[]  FilterDiffOutCoefMin=[]  FilterDiffOutCoefMax=[]  ReciprocalOutMin=[]  ReciprocalOutMax=[]  SumDenOutMin=[]  SumDenOutMax=[]  SumNumOutMin=[]  SumNumOutMax=[]  DivideOutMin=[]  DivideOutMax=[]  UdiffTsProdOutMin=[]  UdiffTsProdOutMax=[]  NTsProdOutMin=[]  NTsProdOutMax=[]  UintegralTsProdOutMin=[]  UintegralTsProdOutMax=[]  UngainTsProdOutMin=[]  UngainTsProdOutMax=[]  ClampingZeroOutDataTypeStr=Inherit: Inherit via back propagation  ClampingZeroOutMin=[]  ClampingZeroOutMax=[]  FilterDenConstantOutDataTypeStr=Inherit: Inherit via back propagation  FilterDenConstantOutMin=[]  FilterDenConstantOutMax=[]  PCopyOutDataTypeStr=Inherit: Inherit via back propagation  PCopyOutMin=[]  PCopyOutMax=[]  NCopyOutDataTypeStr=Inherit: Inherit via back propagation  NCopyOutMin=[]  NCopyOutMax=[]  IntegratorContinuousStateAttributes=''  IntegratorStateMustResolveToSignalObject=off  IntegratorRTWStateStorageClass=Auto  FilterContinuousStateAttributes=''  FilterStateMustResolveToSignalObject=off  FilterRTWStateStorageClass=Auto  ParallelPVariant=InternalParameters  IdealPVariant=Disabled  IVariant=InternalParameters  DVariant=InternalParameters  IntegratorVariant=Continuous  SatVariant=Disabled  AWVariant=Passthrough  PCopyVariant=Disabled  TRVariant=Disabled  FdbkBlocksVariant=Forward  IdealPFdbkVariant=Disabled  SatFdbkVariant=Disabled  DerivativeFilterVariant=ContFilter  NVariant=InternalParameters  NCopyVariant=Disabled  FilterICVariant=InternalICsFilter  IntegratorICVariant=InternalICs  ExternalResetVariant=Disabled  TRSumVariant=Passthrough  SumFdbkVariant=Disabled  SumVariant=Sum_PID  TsampFilterVariant=InternalTs  TsampNgainVariant=Passthrough  TsampIntegralVariant=Disabled_SignalSpec  ExternalSaturationOutDataTypeStr=Inherit: Same as second input
  Sum11 : Sum  Inputs=|+-
  Filtered actuator displacement vector : Outport
  wires:
  PID Controller2/1 -> Mux4/2
  Control Plant4/1 -> Sum11/2, Filtered actuator displacement vector/1  "Filtered actuator displacement vector"
  Demux7/1 -> PID Controller1/1
  Sum11/1 -> Demux7/1
  PID Controller1/1 -> Mux4/1
  Mux4/1 -> Control Plant4/1
  Demux7/2 -> PID Controller2/1
  Target actuator displacement vector (mm)/1 -> Sum11/1

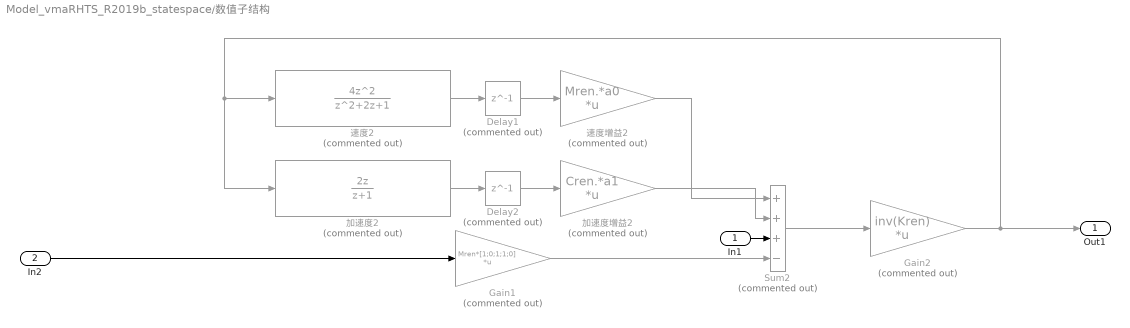
== system Model_vmaRHTS_R2019b_statespace/数值子结构 ==
  In1 : Inport
  In2 : Inport  Port=2
  Delay1 : Delay  Commented=on  DelayLength=1
  Delay2 : Delay  Commented=on  DelayLength=1
  Gain1 : Gain  Commented=on  Gain=Mren*[1;0;1;1;0]  Multiplication=Matrix(K*u)
  Gain2 : Gain  Commented=on  Gain=inv(Kren)  Multiplication=Matrix(K*u)
  Sum2 : Sum  Commented=on  Inputs=+|+|+|-
  加速度2 : DiscreteTransferFcn  Commented=on  Numerator=[2 0]  Denominator=[1 1]
  加速度增益2 : Gain  Commented=on  Gain=Cren.*a1  Multiplication=Matrix(K*u)
  速度2 : DiscreteTransferFcn  Commented=on  Numerator=[4 0 0]  Denominator=[1 2 1]
  速度增益2 : Gain  Commented=on  Gain=Mren.*a0  Multiplication=Matrix(K*u)
  Out1 : Outport
  wires:
  速度增益2/1 -> Sum2/1
  速度2/1 -> Delay1/1
  Gain1/1 -> Sum2/4
  Delay1/1 -> 速度增益2/1
  Delay2/1 -> 加速度增益2/1
  Sum2/1 -> Gain2/1
  加速度增益2/1 -> Sum2/2
  加速度2/1 -> Delay2/1
  Gain2/1 -> Out1/1, 速度2/1, 加速度2/1
  In1/1 -> Sum2/3
  In2/1 -> Gain1/1

== system Model_vmaRHTS_R2019b_statespace/时滞2 ==
  In1 : Inport
  Delay : Delay  DelayLength=j1
  Delay1 : Delay  DelayLength=j2
  Demux2 : Demux  Outputs=2
  Mux4 : Mux  Inputs=2
  Out1 : Outport
  wires:
  In1/1 -> Demux2/1
  Demux2/2 -> Delay1/1
  Delay/1 -> Mux4/1
  Delay1/1 -> Mux4/2
  Demux2/1 -> Delay/1
  Mux4/1 -> Out1/1

== system Model_vmaRHTS_R2019b_statespace/时滞3 ==
  In1 : Inport
  Demux2 : Demux  Outputs=2
  Mux4 : Mux  Inputs=2
  Transport Delay : TransportDelay  DelayTime=1e-3
  Transport Delay1 : TransportDelay  DelayTime=1e-3
  Out1 : Outport
  wires:
  In1/1 -> Demux2/1
  Demux2/2 -> Transport Delay1/1
  Transport Delay/1 -> Mux4/1
  Transport Delay1/1 -> Mux4/2
  Demux2/1 -> Transport Delay/1
  Mux4/1 -> Out1/1

== system Model_vmaRHTS_R2019b_statespace/ 2/Ground motion record ==
  From File : FromFile  FileName=ElCentroAccelNoScaling.mat  SampleTime=dt
  From File1 : FromFile  FileName=KobeAccelNoScaling.mat  SampleTime=dt
  From File2 : FromFile  FileName=MorganAccelNoScaling.mat  SampleTime=dt
  El Centro : Outport
  Kobe : Outport  Port=2
  Morgan : Outport  Port=3
  wires:
  From File/1 -> El Centro/1
  From File2/1 -> Morgan/1
  From File1/1 -> Kobe/1

== system Model_vmaRHTS_R2019b_statespace/ 4/Ground motion record ==
  From File : FromFile  FileName=ElCentroAccelNoScaling.mat  SampleTime=dt
  From File1 : FromFile  FileName=KobeAccelNoScaling.mat  SampleTime=dt
  From File2 : FromFile  FileName=MorganAccelNoScaling.mat  SampleTime=dt
  El Centro : Outport
  Kobe : Outport  Port=2
  Morgan : Outport  Port=3
  wires:
  From File/1 -> El Centro/1
  From File2/1 -> Morgan/1
  From File1/1 -> Kobe/1

== matlab function Model_vmaRHTS_R2019b_statespace/ 数值子结构/MATLAB Function1 ==
  data: U27_MA output; V27_MA output; A27_MA output; Theta21_MA output; VTheta21_MA output; ATheta21_MA output; Theta29_MA output; VTheta29_MA output; ATheta29_MA output; U2nd output; Theta2nd output; U3rd output; Theta3rd output; U1 output; Vel1 output; Acc1 output; accel_grd input; FB_force27 input; FB_moment29 input; FB_moment21 input; Kbar_inv input; MNrt input; CNrt input; Ag input; l input; Rbar input; F input; U0 input; Vel0 input; Acc0 input; a0 parameter; a1 parameter; a2 parameter; a3 parameter; a4 parameter; a5 parameter; a6 parameter; a7 parameter
function [U27_MA,V27_MA,A27_MA,Theta21_MA,VTheta21_MA,ATheta21_MA,Theta29_MA,VTheta29_MA,ATheta29_MA,U2nd,Theta2nd,U3rd,Theta3rd,U1,Vel1,Acc1]=...
    fcn(accel_grd,FB_force27,FB_moment29,FB_moment21,Kbar_inv, MNrt, CNrt,Ag,l,Rbar,F,...
    U0,Vel0,Acc0, a0, a1, a2, a3, a4, a5, a6, a7)
             
             
    % ============================
	% *  Update next iteration   *
	% ============================
    ndof = length(Kbar_inv);
    U1   = zeros(ndof,1);
    Vel1 = zeros(ndof,1);
    Acc1 = zeros(ndof,1);
    
    U27_MA = 0;
    V27_MA = 0;
    A27_MA = 0;

    Theta21_MA = 0;
    VTheta21_MA = 0;
    ATheta21_MA = 0;
% 
%     U6_MA = 0;
%     V6_MA = 0;
%     A6_MA = 0;
    U2nd = 0 ;              %Displacement 2nd story, node 12, DOF 26
    Theta2nd = 0;          %Rotation 2nd story, node 12, DOF 22
    U3rd = 0;              %Displacement 3rd story, node 16, DOF 13
    Theta3rd = 0;           %Rotation 3rd story, node 16, DOF 3


    Theta29_MA = 0;
    VTheta29_MA = 0;
    ATheta29_MA = 0;

    % ============================
	% *  Feedback Force / Moment *
	% ============================
    F(27) = FB_force27;
    F(21) = FB_moment21;
    F(29) = FB_moment29;

    % ==========================
	% *     Update Matrices    *
	% ==========================
    Ag(:)  = accel_grd * l;
    
   	% ==========================
	% * 	  Form Rbar  	   *
	% ==========================
	Rbar = ( (MNrt * ((a0*U0)+(a2*Vel0)+(a3*Acc0))) + ...
		     (CNrt * ((a1*U0)+(a4*Vel0)+(a5*Acc0))) - F - (MNrt * Ag) );
    
    % ==========================
	% * Solve for Displacement *
	% ==========================
	U1 = Kbar_inv * Rbar;
    
	% ============================
	% * Compute Velocity & Accel *
	% ============================
	Acc1=a0*(U1-U0)-a2*Vel0-a3*Acc0;
	Vel1=Vel0+a7*Acc1+a6*Acc0; 

	% ============================
	% *    Output u1 and theta   *
	% ============================
    U27_MA    = U1(27);
    V27_MA    = Vel1(27);
    A27_MA    = Acc1(27);    

%     U6_MA    = U1(27);
%     V6_MA    = Vel1(27);
%     A6_MA    = Acc1(27);

    Theta21_MA = U1(21);
    VTheta21_MA = Vel1(21);
    ATheta21_MA = Acc1(21);

    Theta29_MA = U1(29);
    VTheta29_MA = Vel1(29);
    ATheta29_MA = Acc1(29);
    
    % ADDED by Johnny
    U2nd = U1(26);              %Displacement 2nd story, node 12, DOF 26
    Theta2nd = U1(22);          %Rotation 2nd story, node 12, DOF 22
    U3rd = U1(13);              %Displacement 3rd story, node 16, DOF 13
    Theta3rd = U1(3);           %Rotation 3rd story, node 16, DOF 3

end

== matlab function Model_vmaRHTS_R2019b_statespace/ 数值子结构1/MATLAB Function1 ==
  data: U27_MA output; V27_MA output; A27_MA output; Theta21_MA output; VTheta21_MA output; ATheta21_MA output; Theta29_MA output; VTheta29_MA output; ATheta29_MA output; U2nd output; Theta2nd output; U3rd output; Theta3rd output; U1 output; Vel1 output; Acc1 output; accel_grd input; FB_force27 input; FB_moment29 input; FB_moment21 input; Kbar_inv input; MNrt input; CNrt input; Ag input; l input; Rbar input; F input; U0 input; Vel0 input; Acc0 input; a0 parameter; a1 parameter; a2 parameter; a3 parameter; a4 parameter; a5 parameter; a6 parameter; a7 parameter
function [U27_MA,V27_MA,A27_MA,Theta21_MA,VTheta21_MA,ATheta21_MA,Theta29_MA,VTheta29_MA,ATheta29_MA,U2nd,Theta2nd,U3rd,Theta3rd,U1,Vel1,Acc1]=...
    fcn(accel_grd,FB_force27,FB_moment29,FB_moment21,Kbar_inv, MNrt, CNrt,Ag,l,Rbar,F,...
    U0,Vel0,Acc0, a0, a1, a2, a3, a4, a5, a6, a7)
             
             
    % ============================
	% *  Update next iteration   *
	% ============================
    ndof = length(Kbar_inv);
    U1   = zeros(ndof,1);
    Vel1 = zeros(ndof,1);
    Acc1 = zeros(ndof,1);
    
    U27_MA = 0;
    V27_MA = 0;
    A27_MA = 0;

    Theta21_MA = 0;
    VTheta21_MA = 0;
    ATheta21_MA = 0;
% 
%     U6_MA = 0;
%     V6_MA = 0;
%     A6_MA = 0;
    U2nd = 0 ;              %Displacement 2nd story, node 12, DOF 26
    Theta2nd = 0;          %Rotation 2nd story, node 12, DOF 22
    U3rd = 0;              %Displacement 3rd story, node 16, DOF 13
    Theta3rd = 0;           %Rotation 3rd story, node 16, DOF 3


    Theta29_MA = 0;
    VTheta29_MA = 0;
    ATheta29_MA = 0;

    % ============================
	% *  Feedback Force / Moment *
	% ============================
    F(27) = FB_force27;
    F(21) = FB_moment21;
    F(29) = FB_moment29;

    % ==========================
	% *     Update Matrices    *
	% ==========================
    Ag(:)  = accel_grd * l;
    
   	% ==========================
	% * 	  Form Rbar  	   *
	% ==========================
	Rbar = ( (MNrt * ((a0*U0)+(a2*Vel0)+(a3*Acc0))) + ...
		     (CNrt * ((a1*U0)+(a4*Vel0)+(a5*Acc0))) - F - (MNrt * Ag) );
    
    % ==========================
	% * Solve for Displacement *
	% ==========================
	U1 = Kbar_inv * Rbar;
    
	% ============================
	% * Compute Velocity & Accel *
	% ============================
	Acc1=a0*(U1-U0)-a2*Vel0-a3*Acc0;
	Vel1=Vel0+a7*Acc1+a6*Acc0; 

	% ============================
	% *    Output u1 and theta   *
	% ============================
    U27_MA    = U1(27);
    V27_MA    = Vel1(27);
    A27_MA    = Acc1(27);    

%     U6_MA    = U1(27);
%     V6_MA    = Vel1(27);
%     A6_MA    = Acc1(27);

    Theta21_MA = U1(21);
    VTheta21_MA = Vel1(21);
    ATheta21_MA = Acc1(21);

    Theta29_MA = U1(29);
    VTheta29_MA = Vel1(29);
    ATheta29_MA = Acc1(29);
    
    % ADDED by Johnny
    U2nd = U1(26);              %Displacement 2nd story, node 12, DOF 26
    Theta2nd = U1(22);          %Rotation 2nd story, node 12, DOF 22
    U3rd = U1(13);              %Displacement 3rd story, node 16, DOF 13
    Theta3rd = U1(3);           %Rotation 3rd story, node 16, DOF 3

end
